simulink subsystem "RWDynamics"  (R2021a)
settings: Solver=VariableStepAuto  StartTime=0.0  StopTime=10.0  RelTol=1e-3
values from neighbouring files (symbols this model uses):
  Irw = [5.02e-5, 0, 0; 0, 9.41e-5, 0; 0, 0, 5.02e-5]    [aocs_sim.m]
libraries: vrlib x2
settings Model: Creator=Laura  LastModifiedBy=Laura

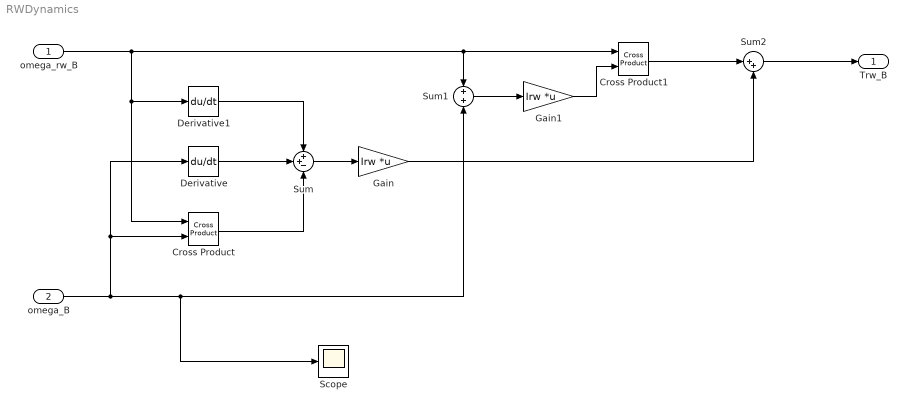
== system RWDynamics ==
  omega_rw_B : Inport
  omega_B : Inport  Port=2
  Cross Product : vrlib/Utilities/Cross Product
  Cross Product1 : vrlib/Utilities/Cross Product
  Derivative : Derivative
  Derivative1 : Derivative
  Gain : Gain  Gain=Irw  Multiplication=Matrix(K*u)
  Gain1 : Gain  Gain=Irw  Multiplication=Matrix(K*u)
  Scope : Scope
  Sum : Sum  Inputs=++-
  Sum1 : Sum
  Sum2 : Sum  Inputs=|++
  Trw_B : Outport
  wires:
  Cross Product1/1 -> Sum2/1
  Gain1/1 -> Cross Product1/2
  Gain/1 -> Sum2/2
  Derivative/1 -> Sum/2
  Sum/1 -> Gain/1
  Cross Product/1 -> Sum/3
  Derivative1/1 -> Sum/1
  Sum1/1 -> Gain1/1
  omega_rw_B/1 -> Cross Product1/1, Sum1/1, Cross Product/1, Derivative1/1
  omega_B/1 -> Derivative/1, Cross Product/2, Scope/1, Sum1/2
  Sum2/1 -> Trw_B/1
